simulink model "ex3"  (R2022b)
settings: Solver=FixedStepAuto  StartTime=0.0  StopTime=20  FixedStep=0.0001  RelTol=1e-3
undefined symbols (not defined in the file or in its folder): Kp, Td, Ti
settings Model: Creator=MPatr  LastModifiedBy=MPatr

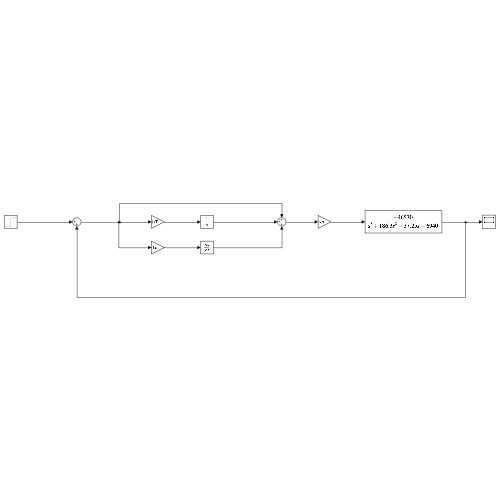
[thumbnail: Simulink's stored preview of the top-level diagram]
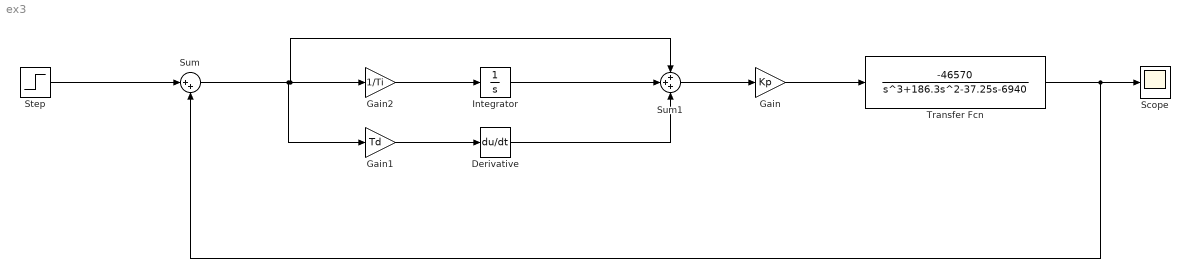
== system ex3 ==
  Derivative : Derivative
  Gain : Gain  Gain=Kp
  Gain1 : Gain  Gain=Td
  Gain2 : Gain  Gain=1/Ti
  Integrator : Integrator
  Scope : Scope
  Step : Step  Time=0  After=2  SampleTime=0
  Sum : Sum  Inputs=|++
  Sum1 : Sum  Inputs=+++
  Transfer Fcn : TransferFcn  Numerator=[-46570]  Denominator=[1 186.3 -37.25 -6940]
  wires:
  Transfer Fcn/1 -> Sum/2, Scope/1
  Step/1 -> Sum/1
  Sum/1 -> Gain1/1, Sum1/1, Gain2/1
  Gain1/1 -> Derivative/1
  Derivative/1 -> Sum1/3
  Gain2/1 -> Integrator/1
  Gain/1 -> Transfer Fcn/1
  Sum1/1 -> Gain/1
  Integrator/1 -> Sum1/2
